simulink model "sampleModel1773"  (R2023a)
settings: Solver=VariableStepAuto  StartTime=0.0  StopTime=10.0  RelTol=1e-3
libraries: hdlsllib x6, simulink x3
settings Model: Creator=user1  LastModifiedBy=user1

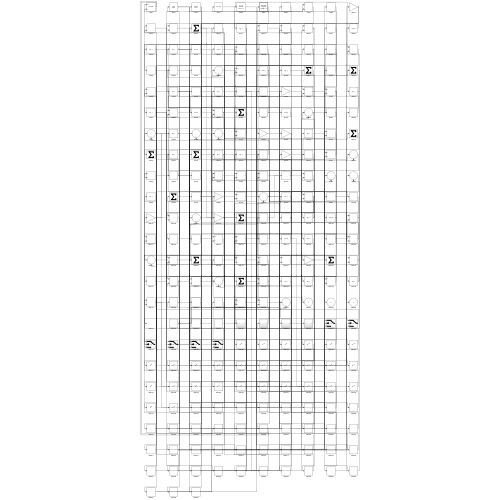
[thumbnail: Simulink's stored preview of the top-level diagram]
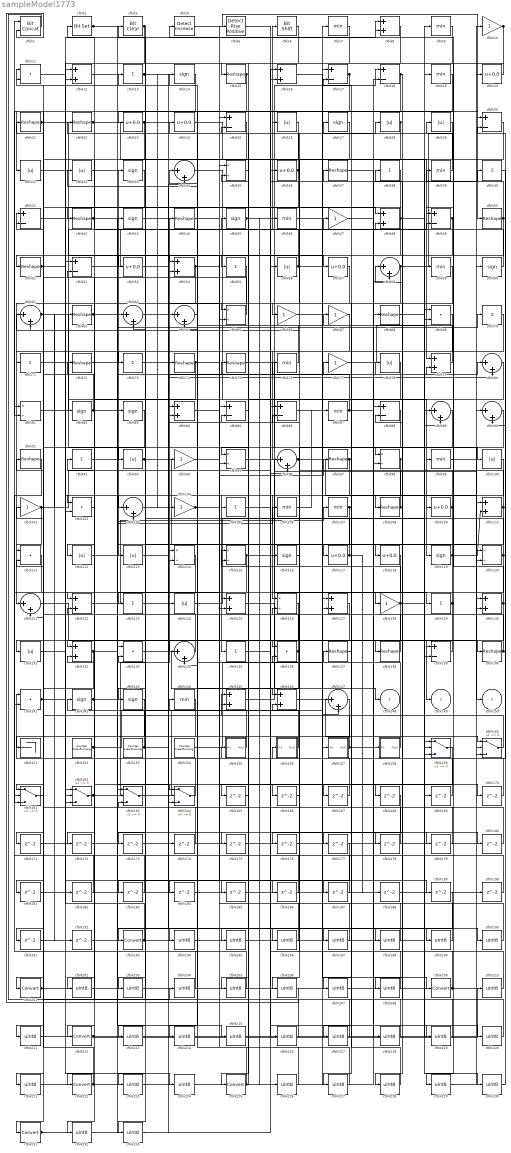
== system sampleModel1773 ==
  cfblk1 : hdlsllib/Logic and Bit Operations/Bit Concat  numInputs=2
  cfblk{10,47,66..67,77,94,101,104,128} (9 alike) : Gain
  cfblk{26,28..29,31..32,56,78,93,100,112..113,124,131} (13 alike) : Abs  SaturateOnIntegerOverflow=off
  cfblk{11,69,102,111,133,136,141} (7 alike) : DotProduct  OutDataTypeStr=Inherit: Inherit via internal rule
  cfblk{34,58,61,63..64,80,89..90,96,103,121,134,147} (13 alike) : Sum  Inputs=|++
  cfblk{13,38,40,55,70..71,73,92,105,123,129,135} (12 alike) : Sum  Inputs=+
  cfblk{7,9,19,39,46,59,76,87,99,106..107,144} (12 alike) : MinMax
  cfblk{15,21..22,37,42,44,50..51,62,68,72,74..75,91,97,108,137..138,140} (19 alike) : Reshape
  cfblk{20,23..24,36,53,57,109,117..118} (9 alike) : Bias  Bias=0.0  SaturateOnIntegerOverflow=off
  cfblk{8,12,16,48,54,79,84,110,122,125,127,130,132,145..146} (15 alike) : Sum
  cfblk{35,65,81,95,98,114..115,120,126} (9 alike) : Product  Inputs=*/  RndMeth=Zero  SaturateOnIntegerOverflow=on
  cfblk{14,27,33,43,45,60,82..83,116,119,142..143} (12 alike) : Signum
  cfblk{17..18,25,30,41,49,52,85..86,88,139} (11 alike) : Sum  Inputs=+-
  cfblk151 : Terminator
  cfblk152 : hdlsllib/Sources/Counter Free-Running  NumBits=16  tsamp=-1
  cfblk153 : hdlsllib/Sources/Counter Free-Running  NumBits=16  tsamp=-1
  cfblk154 : hdlsllib/Sources/Counter Free-Running  NumBits=16  tsamp=-1
  cfblk155 : Subsystem
      settings: LibrarySourceBlock=|
      | hdlsllib/Ports &
      | Subsystems/Subsystem
  cfblk156 : Subsystem
      settings: LibrarySourceBlock=|
      | hdlsllib/Ports &
      | Subsystems/Subsystem
  cfblk157 : Subsystem
      settings: LibrarySourceBlock=|
      | hdlsllib/Ports &
      | Subsystems/Subsystem
  cfblk158 : Subsystem
      settings: LibrarySourceBlock=|
      | hdlsllib/Ports &
      | Subsystems/Subsystem
  cfblk{159..164} (6 alike) : Switch  SaturateOnIntegerOverflow=off  InputSameDT=off
  cfblk{165..192} (28 alike) : Delay  SampleTime=1
  cfblk{193,201,209,212,222,225,231} (7 alike) : DataTypeConversion  SaturateOnIntegerOverflow=off  RndMeth=Floor
  cfblk{194..200,202..208,210..211,213..221,223..224,226..230,232..233} (34 alike) : DataTypeConversion  OutDataTypeStr=uint8  SaturateOnIntegerOverflow=off  RndMeth=Floor
  cfblk2 : simulink/Logic and Bit Operations/Bit Set  iBit=0
      settings: LibrarySourceBlock=|
      | hdlsllib/Logic and Bit
      | Operations/Bit Set
  cfblk3 : simulink/Logic and Bit Operations/Bit Clear  iBit=0
      settings: LibrarySourceBlock=|
      | hdlsllib/Logic and Bit
      | Operations/Bit Clear
  cfblk4 : simulink/Logic and Bit Operations/Detect Increase  vinit=0.0  OutDataTypeStr=boolean
      settings: LibrarySourceBlock=|
      | hdlsllib/Logic and Bit
      | Operations/Detect
      | Increase
  cfblk5 : hdlsllib/Logic and Bit Operations/Detect Rise Positive  vinit=0  OutDataTypeStr=boolean
  cfblk6 : hdlsllib/Logic and Bit Operations/Bit Shift  mode=Shift Left Logical  N=0
  cfblk148 : Outport  VectorParamsAs1DForOutWhenUnconnected=off
  cfblk149 : Outport  Port=2  VectorParamsAs1DForOutWhenUnconnected=off
  cfblk150 : Outport  Port=3  VectorParamsAs1DForOutWhenUnconnected=off
  wires:
  cfblk81/1 -> cfblk47/1
  cfblk134/1 -> cfblk44/1
  cfblk19/1 -> cfblk31/1
  cfblk58/1 -> cfblk4/1, cfblk227/1
  cfblk112/1 -> cfblk33/1
  cfblk146/1 -> cfblk160/1
  cfblk45/1 -> cfblk48/2, cfblk226/1
  cfblk106/1 -> cfblk87/1
  cfblk141/1 -> cfblk8/2, cfblk182/1
  cfblk95/1 -> cfblk129/1
  cfblk132/1 -> cfblk70/1, cfblk151/1
  cfblk59/1 -> cfblk121/1
  cfblk162/1 -> cfblk124/1, cfblk106/1
  cfblk122/1 -> cfblk107/1
  cfblk61/1 -> cfblk119/1, cfblk192/1
  cfblk12/1 -> cfblk83/1
  cfblk35/1 -> cfblk225/1
  cfblk24/1 -> cfblk79/1
  cfblk125/1 -> cfblk148/1
  cfblk145/1 -> cfblk18/1
  cfblk4/1 -> cfblk50/1
  cfblk144/1 -> cfblk193/1
  cfblk69/1 -> cfblk212/1
  cfblk100/1 -> cfblk135/1
  cfblk153/1 -> cfblk64/1, cfblk72/1
  cfblk6/1 -> cfblk105/1
  cfblk114/1 -> cfblk231/1
  cfblk93/1 -> cfblk118/1, cfblk49/2
  cfblk36/1 -> cfblk143/1, cfblk2/1, cfblk102/1
  cfblk42/1 -> cfblk57/1, cfblk164/2, cfblk120/2
  cfblk123/1 -> cfblk140/1
  cfblk60/1 -> cfblk6/1
  cfblk155/1(Out1) -> cfblk3/1
  cfblk34/1 -> cfblk109/1
  cfblk7/1 -> cfblk123/1
  cfblk67/1 -> cfblk161/1
  cfblk50/1 -> cfblk39/1, cfblk63/2
  cfblk15/1 -> cfblk54/1, cfblk162/2
  cfblk9/1 -> cfblk73/1
  cfblk142/1 -> cfblk52/2, cfblk200/1
  cfblk2/1 -> cfblk30/1, cfblk197/1
  cfblk55/1 -> cfblk64/2
  cfblk39/1 -> cfblk14/1
  cfblk139/1 -> cfblk131/1
  cfblk113/1 -> cfblk75/1
  cfblk121/1 -> cfblk136/1
  cfblk133/1 -> cfblk146/1
  cfblk65/1 -> cfblk21/1
  cfblk54/1 -> cfblk93/1, cfblk179/1
  cfblk76/1 -> cfblk13/1
  cfblk91/1 -> cfblk161/2
  cfblk107/1 -> cfblk77/1, cfblk173/1
  cfblk117/1 -> cfblk11/1, cfblk188/1
  cfblk158/1(Out1) -> cfblk54/2
  cfblk70/1 -> cfblk96/1
  cfblk98/1 -> cfblk126/1, cfblk102/2
  cfblk129/1 -> cfblk149/1, cfblk125/1
  cfblk147/1 -> cfblk201/1
  cfblk128/1 -> cfblk89/2, cfblk115/1, cfblk203/1
  cfblk78/1 -> cfblk95/1
  cfblk109/1 -> cfblk45/1, cfblk208/1
  cfblk22/1 -> cfblk163/2, cfblk89/1, cfblk99/1
  cfblk154/1 -> cfblk7/1
  cfblk87/1 -> cfblk34/1, cfblk58/2
  cfblk38/1 -> cfblk103/1
  cfblk136/1 -> cfblk122/2, cfblk194/1
  cfblk3/1 -> cfblk12/2, cfblk223/1
  cfblk163/1 -> cfblk46/1
  cfblk75/1 -> cfblk150/1
  cfblk41/1 -> cfblk95/2
  cfblk40/1 -> cfblk155/1(In1)
  cfblk20/1 -> cfblk15/1
  cfblk21/1 -> cfblk113/1, cfblk71/1
  cfblk119/1 -> cfblk110/2, cfblk141/2, cfblk116/1
  cfblk73/1 -> cfblk34/2
  cfblk5/1 -> cfblk138/1
  cfblk77/1 -> cfblk19/1
  cfblk127/1 -> cfblk222/1
  cfblk49/1 -> cfblk178/1, cfblk229/1
  cfblk16/1 -> cfblk209/1
  cfblk52/1 -> cfblk5/1
  cfblk33/1 -> cfblk121/2
  cfblk97/1 -> cfblk185/1, cfblk186/1
  cfblk120/1 -> cfblk27/1, cfblk164/3, cfblk76/1
  cfblk31/1 -> cfblk53/1
  cfblk79/1 -> cfblk32/1
  cfblk74/1 -> cfblk112/1, cfblk79/2
  cfblk152/1 -> cfblk80/1, cfblk40/1
  cfblk140/1 -> cfblk41/1, cfblk30/2
  cfblk110/1 -> cfblk84/1, cfblk139/2
  cfblk156/1(Out1) -> cfblk74/1
  cfblk29/1 -> cfblk55/1
  cfblk131/1 -> cfblk82/1
  cfblk27/1 -> cfblk66/1
  cfblk57/1 -> cfblk65/1
  cfblk138/1 -> cfblk17/2
  cfblk51/1 -> cfblk189/1, cfblk224/1
  cfblk111/1 -> cfblk161/3
  cfblk164/1 -> cfblk141/1
  cfblk48/1 -> cfblk42/1, cfblk181/1, cfblk230/1
  cfblk116/1 -> cfblk26/1
  cfblk160/1 -> cfblk145/1
  cfblk18/1 -> cfblk108/1, cfblk164/1
  cfblk99/1 -> cfblk120/1
  cfblk84/1 -> cfblk98/1
  cfblk115/1 -> cfblk20/1, cfblk162/3
  cfblk30/1 -> cfblk49/1
  cfblk62/1 -> cfblk132/1, cfblk134/1
  cfblk101/1 -> cfblk111/1, cfblk62/1, cfblk37/1
  cfblk72/1 -> cfblk103/2
  cfblk46/1 -> cfblk128/1
  cfblk71/1 -> cfblk158/1(In1)
  cfblk161/1 -> cfblk41/2
  cfblk56/1 -> cfblk157/1(In1), cfblk22/1
  cfblk23/1 -> cfblk80/2, cfblk211/1
  cfblk103/1 -> cfblk94/1
  cfblk11/1 -> cfblk48/1
  cfblk66/1 -> cfblk28/1
  cfblk82/1 -> cfblk78/1, cfblk11/2, cfblk125/2
  cfblk96/1 -> cfblk130/2, cfblk100/1
  cfblk80/1 -> cfblk117/1
  cfblk14/1 -> cfblk51/1
  cfblk28/1 -> cfblk134/2, cfblk184/1
  cfblk102/1 -> cfblk122/1
  cfblk108/1 -> cfblk38/1, cfblk61/2
  cfblk124/1 -> cfblk9/1
  cfblk13/1 -> cfblk65/2, cfblk104/1
  cfblk44/1 -> cfblk8/1
  cfblk157/1(Out1) -> cfblk91/1, cfblk170/1
  cfblk17/1 -> cfblk81/2, cfblk165/1
  cfblk10/1 -> cfblk139/1, cfblk23/1
  cfblk104/1 -> cfblk97/1, cfblk187/1
  cfblk130/1 -> cfblk29/1, cfblk167/1
  cfblk94/1 -> cfblk166/1
  cfblk166/1 -> cfblk146/2
  cfblk167/1 -> cfblk126/2
  cfblk105/1 -> cfblk168/1
  cfblk169/1 -> cfblk52/1
  cfblk170/1 -> cfblk132/2
  cfblk83/1 -> cfblk171/1
  cfblk171/1 -> cfblk96/2
  cfblk25/1 -> cfblk172/1
  cfblk172/1 -> cfblk160/2
  cfblk173/1 -> cfblk110/1
  cfblk53/1 -> cfblk174/1
  cfblk174/1 -> cfblk163/1
  cfblk63/1 -> cfblk175/1
  cfblk89/1 -> cfblk176/1
  cfblk176/1 -> cfblk130/1
  cfblk118/1 -> cfblk177/1
  cfblk178/1 -> cfblk61/1
  cfblk179/1 -> cfblk163/3
  cfblk32/1 -> cfblk180/1
  cfblk180/1 -> cfblk84/2
  cfblk181/1 -> cfblk98/2
  cfblk182/1 -> cfblk162/1
  cfblk8/1 -> cfblk183/1
  cfblk183/1 -> cfblk81/1
  cfblk184/1 -> cfblk159/1
  cfblk185/1 -> cfblk160/3
  cfblk186/1 -> cfblk145/2
  cfblk187/1 -> cfblk115/2
  cfblk188/1 -> cfblk159/2
  cfblk190/1 -> cfblk133/1
  cfblk26/1 -> cfblk191/1
  cfblk191/1 -> cfblk17/1
  cfblk192/1 -> cfblk18/2
  cfblk193/1 -> cfblk25/1, cfblk12/1
  cfblk194/1 -> cfblk144/1
  cfblk85/1 -> cfblk195/1
  cfblk195/1 -> cfblk169/1
  cfblk43/1 -> cfblk196/1
  cfblk196/1 -> cfblk85/1
  cfblk197/1 -> cfblk85/2
  cfblk86/1 -> cfblk198/1
  cfblk198/1 -> cfblk156/1(In1)
  cfblk37/1 -> cfblk199/1
  cfblk199/1 -> cfblk86/1
  cfblk200/1 -> cfblk86/2
  cfblk201/1 -> cfblk63/1, cfblk59/1
  cfblk143/1 -> cfblk202/1
  cfblk202/1 -> cfblk147/1
  cfblk203/1 -> cfblk147/2
  cfblk1/1 -> cfblk204/1
  cfblk204/1 -> cfblk142/1
  cfblk165/1 -> cfblk205/1
  cfblk205/1 -> cfblk1/1
  cfblk168/1 -> cfblk206/1
  cfblk206/1 -> cfblk1/2
  cfblk137/1 -> cfblk207/1
  cfblk207/1 -> cfblk10/1
  cfblk208/1 -> cfblk137/1
  cfblk209/1 -> cfblk58/1, cfblk136/2
  cfblk210/1 -> cfblk16/1
  cfblk211/1 -> cfblk16/2
  cfblk212/1 -> cfblk210/1, cfblk159/3, cfblk60/1
  cfblk177/1 -> cfblk213/1
  cfblk213/1 -> cfblk69/1
  cfblk64/1 -> cfblk214/1
  cfblk214/1 -> cfblk69/2
  cfblk92/1 -> cfblk215/1
  cfblk215/1 -> cfblk190/1
  cfblk135/1 -> cfblk216/1
  cfblk216/1 -> cfblk92/1
  cfblk88/1 -> cfblk217/1
  cfblk217/1 -> cfblk133/2
  cfblk47/1 -> cfblk218/1
  cfblk218/1 -> cfblk88/1
  cfblk175/1 -> cfblk219/1
  cfblk219/1 -> cfblk88/2
  cfblk68/1 -> cfblk220/1
  cfblk220/1 -> cfblk101/1
  cfblk126/1 -> cfblk221/1
  cfblk221/1 -> cfblk68/1
  cfblk222/1 -> cfblk111/2, cfblk36/1
  cfblk223/1 -> cfblk127/1
  cfblk224/1 -> cfblk127/2
  cfblk225/1 -> cfblk25/2, cfblk24/1
  cfblk226/1 -> cfblk35/1
  cfblk227/1 -> cfblk35/2
  cfblk90/1 -> cfblk228/1
  cfblk228/1 -> cfblk67/1
  cfblk229/1 -> cfblk90/1
  cfblk230/1 -> cfblk90/2
  cfblk231/1 -> cfblk56/1, cfblk43/1
  cfblk159/1 -> cfblk232/1
  cfblk232/1 -> cfblk114/1
  cfblk189/1 -> cfblk233/1
  cfblk233/1 -> cfblk114/2

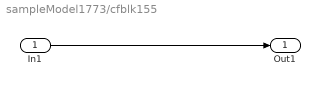
== system sampleModel1773/cfblk155 ==
  In1 : Inport
  Out1 : Outport
  wires:
  In1/1 -> Out1/1

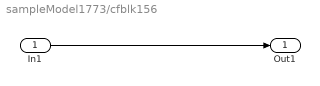
== system sampleModel1773/cfblk156 ==
  In1 : Inport
  Out1 : Outport
  wires:
  In1/1 -> Out1/1

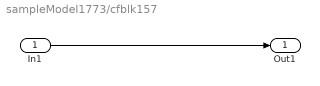
== system sampleModel1773/cfblk157 ==
  In1 : Inport
  Out1 : Outport
  wires:
  In1/1 -> Out1/1

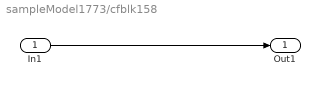
== system sampleModel1773/cfblk158 ==
  In1 : Inport
  Out1 : Outport
  wires:
  In1/1 -> Out1/1
